simulink model "bd_ess_test"  (Simulink 3.00)
settings: Solver=ode1  SolverMode=SingleTasking  StartTime=0.0  StopTime=inf  FixedStep=1  RelTol=1e-3  AbsTol=1e-6
libraries: lib_energy_storage x1
settings Model: LastModifiedBy=tmarkel

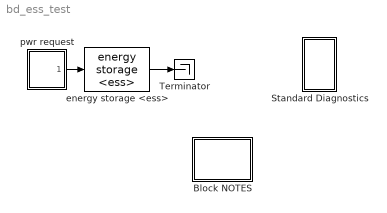
== system bd_ess_test ==
  Block NOTES : Subsystem
      mask Display: disp('Block\nNOTES')
  Standard Diagnostics : Subsystem
  Terminator : Terminator
  energy storage <ess> : lib_energy_storage/energy storage <ess>
  pwr request : Subsystem  mask(Repeating table){@1=ess_pwr_req(:,1), @2=ess_pwr_req(:,2)}
      mask prompts: @1 "Time values:"; @2 "Output values:"
      mask help:
      | Repeating table.
      | Enter values of time and output for first cycle.
      mask init:
      | period = max(@1); t = @1; y = @2;
      mask Help: Repeats cycle given in table. Time values should be monotonically increasing.
  wires:
  pwr request/1(out_1) -> energy storage <ess>/1
  energy storage <ess>/1 -> Terminator/1

== system bd_ess_test/Block NOTES ==
  note: This model is used with the btry_specs.m script file to determine the discharge power,
      | charge power and energy capacity for a single battery module.
      |  The model is linked to the internal resistance model in the
      | lib_energy_storage.mdl library. (tm:07/24/01)

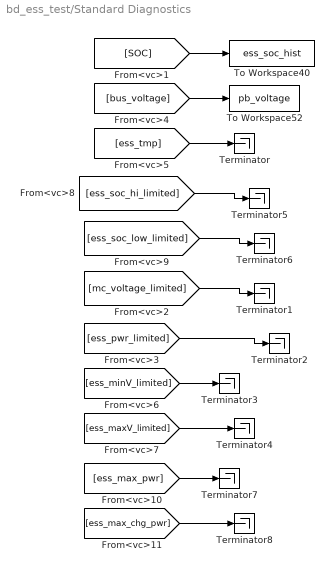
== system bd_ess_test/Standard Diagnostics ==
  Terminator{,1..8} (9 alike) : Terminator
  To Workspace40 : ToWorkspace  VariableName=ess_soc_hist  SampleTime=-1  SaveFormat=Matrix
  To Workspace52 : ToWorkspace  VariableName=pb_voltage  SampleTime=-1  SaveFormat=Matrix
  wires:
  [SOC] -> To Workspace40/1
  [ess_maxV_limited] -> Terminator4/1
  [ess_soc_low_limited] -> Terminator6/1
  [ess_minV_limited] -> Terminator3/1
  [ess_pwr_limited] -> Terminator2/1
  [mc_voltage_limited] -> Terminator1/1
  [bus_voltage] -> To Workspace52/1
  [ess_tmp] -> Terminator/1
  [ess_soc_hi_limited] -> Terminator5/1
  [ess_max_chg_pwr] -> Terminator8/1
  [ess_max_pwr] -> Terminator7/1

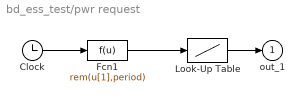
== system bd_ess_test/pwr request ==
  Clock : Clock
      settings: DisplayTime=off  Decimation=10
  Fcn1 : Fcn  Expr=rem(u[1],period)
  Look-Up Table : Lookup  InputValues=t  OutputValues=y
  out_1 : Outport  Port=1  InitialOutput=0
  wires:
  Look-Up Table/1 -> out_1/1
  Clock/1 -> Fcn1/1
  Fcn1/1 -> Look-Up Table/1
